simulink model "EREV_1_Model_RL"  (R2025a)
settings: Solver=ode4  StartTime=0.0  StopTime=1369  FixedStep=0.05  MaxStep=0.01  RelTol=1e-3
undefined symbols (not defined in the file): Af, bsfc_map, Cd, eff_map_F, eff_map_R, eff_spd_F_rpm, eff_spd_R_rpm, eff_trq_F, eff_trq_R, eng_speed_bsfc, eng_speed_rpm, eng_sweet_spot_speed, eng_sweet_spot_torque, eng_torque_bsfc, eng_torque_curve, f_roll, g, G_final_F, G_final_R_1st, G_final_R_2nd, M_veh, Q_bat_Ah, Q_bat_kWh, R_int_base, R_multiplier, r_tire, rho, shift_duration, SOC_init, SOC_R_table, T_brake_max, T_motor_F_curve, T_motor_R_curve, T_motor_R_max, T_wheel_brake_max, T_wheel_max_current, tau_m_F, tau_m_R, theta, torque_split_F_4wd, torque_split_R_4wd, V_downshift_kph, v_regen_min, V_upshift_kph, VOC_map, VOC_SOC, Vt_init, w_motor_F_rpm, w_motor_R_rpm
libraries: simulink x2, autolibshared x1, slpidlib x1, rllib x1
(part 2 of 2)

== system EREV_1_Model_RL/VCU/Level 2_TorqueCalculation/Gear_Ratio_Selection ==
  RL_action : Inport
  Constant : Constant  Value=G_final_R_1st
  Constant1 : Constant  Value=G_final_R_2nd
  Constant2 : Constant  Value=0
  MATLAB Function : MATLAB Function  TreatAsAtomicUnit=on  SystemSampleTime=0.05
  Sampling Time (0.01s) : Constant  Value=0.05
  Switch : Switch  Criteria=u2 > Threshold  Threshold=0.5  SaturateOnIntegerOverflow=off  InputSameDT=off
  Switch1 : Switch  Criteria=u2 > Threshold  Threshold=1.5  SaturateOnIntegerOverflow=off  InputSameDT=off
  To Workspace : ToWorkspace  VariableName=Shift_In_Progress  SaveFormat=Timeseries  SampleTime=-1
  To Workspace1 : ToWorkspace  VariableName=Gear_R  SaveFormat=Timeseries  SampleTime=-1
  shift_duration (0.3s) : Constant  Value=shift_duration
  G_final_R : Outport
  Gear_R : Outport  Port=2
  tag scope: Gear_R=global, Gear_log=global, Shift_In_Progress=global
  wires:
  Constant/1 -> Switch1/3
  Constant1/1 -> Switch1/1
  Switch/1 -> G_final_R/1
  Sampling Time (0.01s)/1 -> MATLAB Function/2(Ts)
  shift_duration (0.3s)/1 -> MATLAB Function/3(shift_duration)
  MATLAB Function/2(Shift_In_Progress) -> To Workspace/1, [Shift_In_Progress]
  Constant2/1 -> Switch/3
  Switch1/1 -> Switch/1
  RL_action/1 -> MATLAB Function/1(Target_Gear)
  MATLAB Function/1(Gear_Actual) -> To Workspace1/1, [Gear_log], [Gear_R], Gear_R/1, Switch1/2, Switch/2

== system EREV_1_Model_RL/VCU/Level 2_TorqueCalculation/Pedal_to_Wheel_Torque ==
  Ap : Inport
  Bp : Inport  Port=2
  G_final_R : Inport  Port=3
  Gain1 : Gain  Gain=T_wheel_brake_max
  Gain2 : Gain  Gain=T_motor_R_max
  Product : Product
  T_wheel_prop : Outport
  T_wheel_brake : Outport  Port=2
  wires:
  Bp/1 -> Gain1/1
  Ap/1 -> Gain2/1
  Gain1/1 -> T_wheel_brake/1
  Product/1 -> T_wheel_prop/1
  Gain2/1 -> Product/2
  G_final_R/1 -> Product/1

== system EREV_1_Model_RL/VCU/Level3_Distribution&Limitation/Front_Rear_Distribution ==
  Mode_F : Inport
  T_wh eel_prop : Inport  Port=2
  G_final_R : Inport  Port=3
  Constant1 : Constant
  Constant2 : Constant  Value=0
  Divide1 : Product  Inputs=/*
  Divide2 : Product  Inputs=*/
  Gain : Gain  Gain=torque_split_R_4wd
  Gain1 : Gain  Gain=torque_split_F_4wd
  Gain2 : Gain  Gain=1/G_final_F
  Relational Operator : RelationalOperator  Operator===  OutDataTypeStr=boolean  RndMeth=Simplest  InputSameDT=off
  Switch : Switch  Criteria=u2 ~= 0  SaturateOnIntegerOverflow=off  InputSameDT=off
  Switch1 : Switch  Criteria=u2 ~= 0  SaturateOnIntegerOverflow=off  InputSameDT=off
  Tprop_F_d : Outport
  Tprop_R_d : Outport  Port=2
  wires:
  T_wh eel_prop/1 -> Gain/1, Gain1/1, Divide1/2  "Tprop_motor_d"
  Mode_F/1 -> Relational Operator/2
  Constant1/1 -> Relational Operator/1
  Relational Operator/1 -> Switch/2, Switch1/2
  Constant2/1 -> Switch/3
  Switch/1 -> Tprop_F_d/1
  Divide2/1 -> Switch1/1
  Gain/1 -> Divide2/1
  G_final_R/1 -> Divide2/2, Divide1/1
  Gain1/1 -> Gain2/1
  Gain2/1 -> Switch/1
  Divide1/1 -> Switch1/3
  Switch1/1 -> Tprop_R_d/1

== system EREV_1_Model_RL/VCU/Level3_Distribution&Limitation/RegenFriction_Distribution_v2 ==
  T_wheel_brake : Inport
  Vel_kph : Inport  Port=2
  SOC : Inport  Port=3
  Mode_F : Inport  Port=4
  G_final_R : Inport  Port=5
  Regen/Friction_Distribution Matlab Function : MATLAB Function  TreatAsAtomicUnit=on
  Scope : Scope  NumInputPorts=4
      settings: ActiveDisplayYMinimum=-1  ActiveDisplayYMaximum=1  DataLoggingVariableName=ScopeData13
  Scope1 : Scope  NumInputPorts=5
      settings: ActiveDisplayYMinimum=-5641.4095969862055  ActiveDisplayYMaximum=772.68637287585079  DataLoggingVariableName=ScopeData14
  T_motor_F_regen_d : Outport
  T_wheel_F_fric_d : Outport  Port=2
  T_motor_R_regen_d : Outport  Port=3
  T_wheel_R_fric_d : Outport  Port=4
  wires:
  G_final_R/1 -> Scope1/5, Regen/Friction_Distribution Matlab Function/5(G_final_R)
  Mode_F/1 -> Scope1/4, Regen/Friction_Distribution Matlab Function/4(Mode_F)
  SOC/1 -> Scope1/3, Regen/Friction_Distribution Matlab Function/3(SOC)
  Vel_kph/1 -> Regen/Friction_Distribution Matlab Function/2(Vel_kph), Scope1/2
  T_wheel_brake/1 -> Scope1/1, Regen/Friction_Distribution Matlab Function/1(T_wheel_brake)  "T_wheel_brake"
  Regen/Friction_Distribution Matlab Function/4(T_wheel_R_fric) -> Scope/4, T_wheel_R_fric_d/1
  Regen/Friction_Distribution Matlab Function/2(T_wheel_F_fric) -> Scope/2, T_wheel_F_fric_d/1
  Regen/Friction_Distribution Matlab Function/1(T_motor_F_regen) -> Scope/1, T_motor_F_regen_d/1
  Regen/Friction_Distribution Matlab Function/3(T_motor_R_regen) -> T_motor_R_regen_d/1, Scope/3

== system EREV_1_Model_RL/VCU/Level4_EngineControl/Engine_Command_Gen ==
  Engine_ON : Inport
  Constant : Constant  Value=eng_sweet_spot_torque
  Constant1 : Constant  Value=0
  Constant2 : Constant  Value=eng_sweet_spot_speed
  Constant3 : Constant  Value=0
  Switch : Switch  Criteria=u2 ~= 0  SaturateOnIntegerOverflow=off  InputSameDT=off
  Switch1 : Switch  Criteria=u2 > Threshold  SaturateOnIntegerOverflow=off  InputSameDT=off
  Engine_Speed_cmd : Outport
  Engine_Torque_cmd : Outport  Port=2
  wires:
  Engine_ON/1 -> Switch1/2, Switch/2
  Switch/1 -> Engine_Speed_cmd/1  "Engine_Speed_cmd"
  Switch1/1 -> Engine_Torque_cmd/1  "Engine_Torque_cmd"
  Constant1/1 -> Switch/3
  Constant3/1 -> Switch1/3
  Constant/1 -> Switch1/1
  Constant2/1 -> Switch/1

== system EREV_1_Model_RL/VCU/Level4_EngineControl/Engine_ONOFF_Logic ==
  Mode_F : Inport
  Constant : Constant  Value=2
  Equal : RelationalOperator  Operator===  OutDataTypeStr=boolean  RndMeth=Simplest  InputSameDT=off
  Engine_ON : Outport
  wires:
  Mode_F/1 -> Equal/1
  Constant/1 -> Equal/2
  Equal/1 -> Engine_ON/1

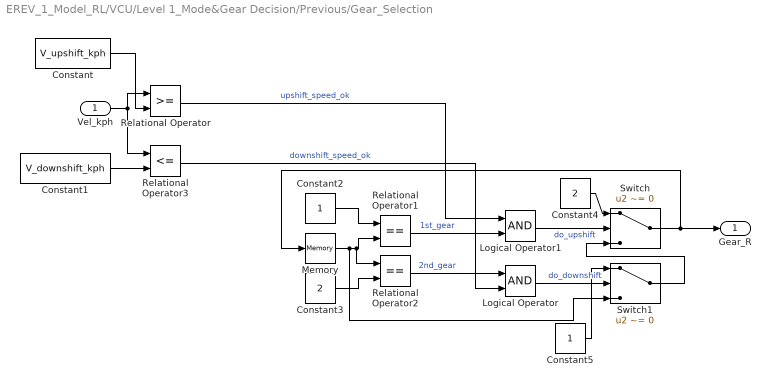
== system EREV_1_Model_RL/VCU/Level 1_Mode&Gear Decision/Previous/Gear_Selection ==
  Vel_kph : Inport
  Constant : Constant  Value=V_upshift_kph
  Constant1 : Constant  Value=V_downshift_kph
  Constant2 : Constant
  Constant3 : Constant  Value=2
  Constant4 : Constant  Value=2
  Constant5 : Constant
  Logical Operator : Logic  AllPortsSameDT=off  OutDataTypeStr=boolean
  Logical Operator1 : Logic  AllPortsSameDT=off  OutDataTypeStr=boolean
  Memory : Memory  InitialCondition=1
  Relational Operator : RelationalOperator  OutDataTypeStr=boolean  RndMeth=Simplest  InputSameDT=off
  Relational Operator1 : RelationalOperator  Operator===  OutDataTypeStr=boolean  RndMeth=Simplest  InputSameDT=off
  Relational Operator2 : RelationalOperator  Operator===  OutDataTypeStr=boolean  RndMeth=Simplest  InputSameDT=off
  Relational Operator3 : RelationalOperator  Operator=<=  OutDataTypeStr=boolean  RndMeth=Simplest  InputSameDT=off
  Switch : Switch  Criteria=u2 ~= 0  SaturateOnIntegerOverflow=off  InputSameDT=off
  Switch1 : Switch  Criteria=u2 ~= 0  SaturateOnIntegerOverflow=off  InputSameDT=off
  Gear_R : Outport
  wires:
  Vel_kph/1 -> Relational Operator/1, Relational Operator3/1
  Constant/1 -> Relational Operator/2
  Constant1/1 -> Relational Operator3/2
  Relational Operator/1 -> Logical Operator1/1  "upshift_speed_ok"
  Relational Operator3/1 -> Logical Operator/2  "downshift_speed_ok"
  Memory/1 -> Switch1/3, Relational Operator2/1, Relational Operator1/2
  Constant2/1 -> Relational Operator1/1
  Constant3/1 -> Relational Operator2/2
  Relational Operator1/1 -> Logical Operator1/2  "1st_gear"
  Relational Operator2/1 -> Logical Operator/1  "2nd_gear"
  Logical Operator1/1 -> Switch/2  "do_upshift"
  Logical Operator/1 -> Switch1/2  "do_downshift"
  Switch1/1 -> Switch/3
  Constant4/1 -> Switch/1
  Constant5/1 -> Switch1/1
  Switch/1 -> Memory/1, Gear_R/1

== system EREV_1_Model_RL/VCU/Level 1_Mode&Gear Decision/Previous/Gear_Selection1 ==
  Vel_kph : Inport
  VCU_mode : Inport  Port=2
  Constant : Constant  Value=V_upshift_kph
  Constant1 : Constant  Value=V_downshift_kph
  MATLAB Function : MATLAB Function  TreatAsAtomicUnit=on  SystemSampleTime=0.01
  Gear_R : Outport
  wires:
  VCU_mode/1 -> MATLAB Function/1(VCU_mode)
  MATLAB Function/1(Gear_R) -> Gear_R/1
  Constant1/1 -> MATLAB Function/4(V_downshift_kph)
  Constant/1 -> MATLAB Function/3(V_upshift_kph)
  Vel_kph/1 -> MATLAB Function/2(Vel_kph)

== system EREV_1_Model_RL/VCU/Level 1_Mode&Gear Decision/Previous/Mode_Selection ==
  sys_mode : Inport
  Ap : Inport  Port=2
  Constant1 : Constant  Value=0
  Constant2 : Constant  Value=2
  Constant3 : Constant
  Constant4 : Constant  Value=0.5
  Logical Operator : Logic  AllPortsSameDT=off  OutDataTypeStr=boolean
  Relational Operator : RelationalOperator  Operator===  OutDataTypeStr=boolean  RndMeth=Simplest  InputSameDT=off
  Relational Operator1 : RelationalOperator  Operator===  OutDataTypeStr=boolean  RndMeth=Simplest  InputSameDT=off
  Relational Operator2 : RelationalOperator  Operator=>  OutDataTypeStr=boolean  RndMeth=Simplest  InputSameDT=off
  Switch : Switch  Criteria=u2 ~= 0  SaturateOnIntegerOverflow=off  InputSameDT=off
  Switch1 : Switch  Criteria=u2 ~= 0  SaturateOnIntegerOverflow=off  InputSameDT=off
  Mode_F : Outport
  wires:
  Ap/1 -> Relational Operator2/1
  sys_mode/1 -> Relational Operator/1, Relational Operator1/2
  Constant2/1 -> Relational Operator1/1, Switch1/1  "Mode_F=2(Generator)"
  Constant1/1 -> Switch/3, Relational Operator/2  "Mode_F=0 (2WD Disconnect)"
  Relational Operator/1 -> Logical Operator/1  "EV_mode"
  Relational Operator1/1 -> Switch1/2  "charge_mode"
  Switch/1 -> Switch1/3
  Logical Operator/1 -> Switch/2
  Constant3/1 -> Switch/1  "Mode_F=1 (4WD Motor)"
  Constant4/1 -> Relational Operator2/2
  Relational Operator2/1 -> Logical Operator/2  "Ap_high"
  Switch1/1 -> Mode_F/1  "Mode_Front"

== system EREV_1_Model_RL/VCU/Level 1_Mode&Gear Decision/Previous/SOC_Monitoring ==
  SOC : Inport
  Constant : Constant  Value=2
  Constant1 : Constant  Value=0
  Memory : Memory
  Switch : Switch  Criteria=u2 > Threshold  Threshold=0.3  SaturateOnIntegerOverflow=off  InputSameDT=off
  Switch1 : Switch  Threshold=0.4  SaturateOnIntegerOverflow=off  InputSameDT=off
  sys_mode : Outport
  wires:
  SOC/1 -> Switch1/2, Switch/2
  Constant/1 -> Switch/3
  Constant1/1 -> Switch1/1
  Memory/1 -> Switch/1
  Switch/1 -> Switch1/3
  Switch1/1 -> Memory/1, sys_mode/1

== matlab function EREV_1_Model_RL/Trash/Engine_Command_Gen/MATLAB Function ==
  data: Engien_ON input; Engine_Speed_cmd output; Engine_Torque_cmd output
function [Engine_Speed_cmd, Engine_Torque_cmd] =Engine_Command_Gen(Engien_ON)

if Engine_ON
    Engine_Speed_cmd=2000;
    Engine_Torque_cmd=150;
else
    Engine_Speed_cmd=0;
    Engine_Torque_cmd=0;
end

== matlab function EREV_1_Model_RL/Trash/RegenFriction_Distribution/MATLAB Function1 ==
  data: Tbrake_motor_d input; Tregen_d output; SOC input; Vel_kph input; Tfric_d output
function [Tregen_d, Tfric_d] = RegenFriction_Distribution(Tbrake_motor_d, SOC, Vel_kph)
    regen_enable = (Vel_kph > 10) && (SOC < 0.9);
    
    if regen_enable
        Tregen_max = 203;
        if SOC > 0.8
            Tregen_max = Tregen_max * 0.5;
        end
        
        Tregen_d = min(Tbrake_motor_d, Tregen_max);
        Tfric_d = Tbrake_motor_d - Tregen_d;
    else
        Tregen_d = 0;
        Tfric_d = Tbrake_motor_d;
    end
end

== matlab function EREV_1_Model_RL/Reward Calculator/Reward_Calculator.m Version B ==
  data: vel input; Reward output; vel_desired input; Shift_In_Progress input; eff_motor_R input
%% Reward_Calculator.m
% Version B: Shift Penalty 있음 (변속 중 페널티)

function Reward = Reward_Calculator(vel, vel_desired, Shift_In_Progress, eff_motor_R)
    % 효율 우선 + 변속 억제
    
    %% 1. 속도 추종
    speed_error = vel_desired - vel;
    R_speed = -0.002 * speed_error^2;
    
    %% 2. 모터 효율
    R_eff = (eff_motor_R - 0.5) * 20;
    
    %% 3. Shift Penalty (변속 중인 동안 페널티!)
    R_shift = 0;
    if Shift_In_Progress > 0.5  % boolean check
        R_shift = -1;
    end
    
    %% 총 Reward
    Reward = (R_speed + R_eff + R_shift) * 0.01;
    
end

== matlab function EREV_1_Model_RL/Trash/Mode_Selection/MATLAB Function ==
  data: sys_mode input; Mode_F output; Ap input
function Mode_F = Mode_Selection(sys_mode, Ap)
    switch sys_mode
        case 0  % EV 모드
            if Ap > 50  % 페달 기준 ✅
                Mode_F = 1;  % 4WD
            else
                Mode_F = 0;  % 2WD
            end
        case 1  % Hybrid
            Mode_F = 1;
        case 2  % Charge
            Mode_F = 2;
    end
end

== matlab function EREV_1_Model_RL/VCU/Level3_Distribution&Limitation/RegenFriction_Distribution_v2/Regen//Friction_Distribution Matlab Function ==
  data: T_wheel_brake input; T_motor_F_regen output; Vel_kph input; SOC input; Mode_F input; G_final_R input; T_wheel_F_fric output; T_motor_R_regen output; T_wheel_R_fric output
function [T_motor_F_regen, T_wheel_F_fric, T_motor_R_regen, T_wheel_R_fric] = ...
    RegenFrictionDistribution(T_wheel_brake, Vel_kph, SOC, Mode_F, G_final_R)
%#codegen
% ========================================================================
% EREV Regenerative & Friction Braking Distribution (수정 버전)
% ========================================================================

%% 파라미터
G_final_F = 7.94;
T_motor_F_max = 264;  % Nm (정격 최대 토크)
T_motor_R_max = 304;  % Nm
P_motor_F_max = 67000;  % W
P_motor_R_max = 91000;  % W

regen_ratio_max = 0.8;  % 정격 토크의 80%까지 회생
brake_regen_ratio_max = 0.7;  % 총 제동의 70%까지 회생 허용

v_regen_min = 8;    % km/h
v_regen_full = 15;  % km/h
regen_max_SOC = 0.9;

torque_split_F_4wd = 0.4;
torque_split_R_4wd = 0.6;

%% Step 1: Mode에 따른 전후륜 토크 분배
if Mode_F == 0
    torque_split_F = 0.0;
    torque_split_R = 1.0;
elseif Mode_F == 1
    torque_split_F = torque_split_F_4wd;
    torque_split_R = torque_split_R_4wd;
else
    torque_split_F = 0.0;
    torque_split_R = 1.0;
end

% 전후륜 휠 제동 토크 (음수)
T_wheel_brake_F = T_wheel_brake * torque_split_F;
T_wheel_brake_R = T_wheel_brake * torque_split_R;

%% Step 2: 회생제동 가능 여부 (속도, SOC 기반)
if Vel_kph < v_regen_min
    vel_factor = 0.0;
elseif Vel_kph < v_regen_full
    vel_factor = (Vel_kph - v_regen_min) / (v_regen_full - v_regen_min);
else
    vel_factor = 1.0;
end

if SOC >= regen_max_SOC
    soc_factor = 0.0;
else
    soc_factor = 1.0;
end

regen_available = vel_factor * soc_factor;

%% Step 3: RPM 계산 및 파워 제한
r_tire = 0.369;  % m
w_wheel = Vel_kph / 3.6 / r_tire;  % rad/s

w_motor_F = w_wheel * G_final_F;
w_motor_R = w_wheel * G_final_R;

%% Step 4: 모터별 회생 최대 토크 계산

% === 전륜 ===
% (1) 정격 토크 제한
T_motor_F_limit_rated = -T_motor_F_max * regen_ratio_max;  % -211 Nm

% (2) 파워 제한
if w_motor_F > 0.1
    T_motor_F_limit_power = -P_motor_F_max / w_motor_F;
else
    T_motor_F_limit_power = T_motor_F_limit_rated;
end

% (3) 최종 한계 = 둘 중 작은 것 (절댓값 기준)
T_motor_F_max_regen = max(T_motor_F_limit_rated, T_motor_F_limit_power);

% === 후륜 ===
T_motor_R_limit_rated = -T_motor_R_max * regen_ratio_max;  % -243 Nm

if w_motor_R > 0.1
    T_motor_R_limit_power = -P_motor_R_max / w_motor_R;
else
    T_motor_R_limit_power = T_motor_R_limit_rated;
end

T_motor_R_max_regen = max(T_motor_R_limit_rated, T_motor_R_limit_power);

%% Step 5: 요구 모터 토크 계산
% 휠 제동 토크 → 모터 토크 변환
T_motor_brake_F_request = T_wheel_brake_F / G_final_F;
T_motor_brake_R_request = T_wheel_brake_R / G_final_R;

%% Step 6: 회생 제동 결정

% (1) 회생 가능 토크 (속도/SOC 고려)
T_motor_F_regen_possible = T_motor_F_max_regen * regen_available;
T_motor_R_regen_possible = T_motor_R_max_regen * regen_available;

% (2) 70% 제한 적용 (요구의 70%까지만)
T_motor_F_regen_70pct = T_motor_brake_F_request * brake_regen_ratio_max;
T_motor_R_regen_70pct = T_motor_brake_R_request * brake_regen_ratio_max;

% (3) 최종 회생 토크 = min(가능, 70%제한, 요구) (절댓값 기준)
% max()는 음수에서 절댓값이 작은 것 선택
T_motor_F_regen = max([T_motor_F_regen_possible, T_motor_F_regen_70pct, T_motor_brake_F_request]);
T_motor_R_regen = max([T_motor_R_regen_possible, T_motor_R_regen_70pct, T_motor_brake_R_request]);

%% Step 7: 마찰 제동 보충
% 회생으로 만드는 휠 토크
T_wheel_F_regen = T_motor_F_regen * G_final_F;
T_wheel_R_regen = T_motor_R_regen * G_final_R;

% 부족분을 마찰 제동으로
T_wheel_F_fric = T_wheel_brake_F - T_wheel_F_regen;
T_wheel_R_fric = T_wheel_brake_R - T_wheel_R_regen;

% 음수 방향으로만 (제동)
T_wheel_F_fric = min(T_wheel_F_fric, 0.0);
T_wheel_R_fric = min(T_wheel_R_fric, 0.0);

%% Step 8: 예외 처리
if regen_available < 0.01
    % 회생 불가능 → 전부 마찰 제동
    T_motor_F_regen = 0.0;
    T_motor_R_regen = 0.0;
    T_wheel_F_fric = T_wheel_brake_F;
    T_wheel_R_fric = T_wheel_brake_R;
end

end

== matlab function EREV_1_Model_RL/Trash/Gear_Selection/MATLAB Function ==
  data: Vel_kph input; Gear_R output; Ap input
function Gear_R = Gear_Selection(Vel_kph, Ap)
    persistent prev_gear;
    if isempty(prev_gear)
        prev_gear = 1;
    end
    
    if Vel_kph >= 60 && prev_gear == 1
        Gear_R = 2;
    elseif Vel_kph <= 55 && prev_gear == 2
        Gear_R = 1;
    elseif Ap > 80 && Vel_kph < 80 && prev_gear == 2
        Gear_R = 1;  % 킥다운
    else
        Gear_R = prev_gear;
    end
    
    prev_gear = Gear_R;
end

== matlab function EREV_1_Model_RL/Trash/Front_Rear_Distribution/MATLAB Function ==
  data: Tprop_motor_d input; Tprop_F_d output; Mode_F input; G_final_R input; Tprop_R_d output
function [Tprop_F_d, Tprop_R_d] = FrontRear_Distribution(Tprop_motor_d, Mode_F, G_final_R)
    G_final_F = 8;
    
    if Mode_F == 1  % 4WD
        % 전후륜 50:50 분배
        T_wheel_total = Tprop_motor_d * G_final_R;
        T_wheel_F = T_wheel_total * 0.5;
        T_wheel_R = T_wheel_total * 0.5;
        
        Tprop_F_d = T_wheel_F / G_final_F;
        Tprop_R_d = T_wheel_R / G_final_R;
    else  % 2WD
        Tprop_F_d = 0;
        Tprop_R_d = Tprop_motor_d;
    end
end

== matlab function EREV_1_Model_RL/VCU/Level 2_TorqueCalculation/Gear_Ratio_Selection/MATLAB Function ==
  data: Target_Gear input; Gear_Actual output; Ts input; shift_duration input; Shift_In_Progress output
function [Gear_Actual, Shift_In_Progress] = ShiftDurationLogic(Target_Gear, Ts, shift_duration)
    % Target_Gear: RL이나 Decoder에서 들어오는 목표 기어 (1 또는 2)
    % Ts: 시뮬레이션 샘플 타임 (예: 0.01s)
    % shift_duration: 변속 소요 시간 (예: 0.3s)
    
    persistent current_gear latched_target_gear shift_timer is_shifting
    
    % 초기화 (최초 실행 시)
    if isempty(current_gear)
        current_gear = 1;          % 초기 기어는 1단으로 가정
        latched_target_gear = 1;   % 목표 기어 초기화
        shift_timer = 0;
        is_shifting = false;
    end
    
    %% 1. 변속 트리거 로직 (Toggle -> Target Comparison)
    % 현재 변속 중이 아니고, 목표 기어가 현재 기어와 다르면 변속 시작
    if (Target_Gear ~= current_gear) && ~is_shifting
        is_shifting = true;
        shift_timer = 0;
        latched_target_gear = Target_Gear; % 목표 기어 확정(Latch)
    end
    
    %% 2. 변속 진행 로직 (시간 지연)
    if is_shifting
        shift_timer = shift_timer + Ts;
        
        % 변속 시간이 지났으면 기어 변경 완료
        if shift_timer >= shift_duration
            current_gear = latched_target_gear; % 기어 변경
            is_shifting = false;
            shift_timer = 0;
        end
    end
    
    %% 3. 최종 출력
    if is_shifting
        Gear_Actual = 0; % 변속 중에는 중립(0) -> 동력 끊김 구현
    else
        Gear_Actual = current_gear; % 변속 완료 시 해당 기어 출력
    end
    
    Shift_In_Progress = is_shifting;
end

== matlab function EREV_1_Model_RL/Trash/Motor_Limit_Check/MATLAB Function ==
  data: Tprop_motor_d input; Tprop_limited output; w_motor_R input
% w_motor_R 입력이 있을 때만 사용
function Tprop_limited = Motor_Limit_Check(Tprop_motor_d, w_motor_R)
    % 속도-토크 특성
    w_spd = [0 300 419 524 628 733 838 943 1047 1152 1257 1361] * (pi/30);
    T_max = [203 203 193 156 129 111 98 85 79 72 65 60];
    
    % 현재 속도에서 최대 토크
    T_motor_max = interp1(w_spd, T_max, w_motor_R, 'linear', 60);
    
    % 제한
    Tprop_limited = min(Tprop_motor_d, T_motor_max);
end

== matlab function EREV_1_Model_RL/Reward Calculator/Reward_Calculator.m Version A ==
  data: vel input; Reward output; vel_desired input; Shift_In_Progress input; eff_motor_R input
%% Reward_Calculator.m
% Version A: Shift Penalty 없음

function Reward = Reward_Calculator(vel, vel_desired, Shift_In_Progress, eff_motor_R)
    % 효율 우선 전략
    
    %% 1. 속도 추종
    speed_error = vel_desired - vel;
    R_speed = -0.002 * speed_error^2;
    
    %% 2. 모터 효율 (핵심!)
    R_eff = (eff_motor_R - 0.5) * 20;
    
    %% 3. Shift Penalty (Version A: 없음)
    R_shift = 0;
    
    %% 총 Reward
    Reward = (R_speed + R_eff + R_shift) * 0.01;
    
end

== matlab function EREV_1_Model_RL/VCU/Level 1_Mode&Gear Decision/MATLAB Function ==
  data: RL_Action input; Target_Gear output; SOC input; Mode_F output; Ap input
%% Action_Decoder.m
function [Target_Gear, Mode_F] = Action_Decoder(RL_Action, SOC, Ap)
    
    persistent is_generating;
    if isempty(is_generating)
        is_generating = false;
    end
    
    %% 1. 변속 제어 (RL)
    Target_Gear = RL_Action;  % 1 or 2
    
    %% 2. 발전 제어 (Rule-based Hysteresis)
    if SOC < 0.30
        is_generating = true;
    end
    
    if SOC >= 0.40
        is_generating = false;
    end
    
    if is_generating
        Mode_F = 2;  % 발전
    else
        if Ap > 0.5
            Mode_F = 1;  % 4WD
        else
            Mode_F = 0;  % 2WD
        end
    end
end

== matlab function EREV_1_Model_RL/VCU/Level 1_Mode&Gear Decision/Previous/Gear_Selection1/MATLAB Function ==
  settings: updateMethod=DISCRETE
  data: VCU_mode input; Gear_R output; Vel_kph input; V_upshift_kph input; V_downshift_kph input
function Gear_R = GearSelection(VCU_mode, Vel_kph, V_upshift_kph, V_downshift_kph)
    % VCU_mode: 1=2단변속, 2=1단고정, 3=2단고정
    % Vel_kph: 차량 속도
    % V_upshift_kph: 업시프트 속도 (35)
    % V_downshift_kph: 다운시프트 속도 (30)
    
    persistent current_gear
    
    % 초기화
    if isempty(current_gear)
        current_gear = 1;
    end
    
    % VCU 모드에 따른 기어 선택
    if VCU_mode == 2
        % 1단 고정
        Gear_R = 1;
        current_gear = 1;  % persistent 변수도 업데이트
        
    elseif VCU_mode == 3
        % 2단 고정
        Gear_R = 2;
        current_gear = 2;
        
    else
        % VCU_mode == 1: 2단 변속 (기존 로직)
        
        % 업시프트 (1단 → 2단)
        if current_gear == 1 && Vel_kph >= V_upshift_kph
            current_gear = 2;
        end
        
        % 다운시프트 (2단 → 1단)
        if current_gear == 2 && Vel_kph <= V_downshift_kph
            current_gear = 1;
        end
        
        Gear_R = current_gear;
    end
end
